simulink model "SeatHeaterapp"  (R2015a)
settings: Solver=FixedStepDiscrete  StartTime=0.0  StopTime=10.0  RelTol=1e-3
settings Model: Creator=Morya  LastModifiedBy=Morya
settings DataIOCC: SaveFormat=StructureWithTime
settings OptimizationCC: ZeroExternalMemoryAtStartup=off  ZeroInternalMemoryAtStartup=off  OptimizeModelRefInitCode=on  LifeSpan=1
settings ModelReferenceCC: ModelReferenceNumInstancesAllowed=Single
settings RTWCC: SystemTargetFile=autosar.tlc  GenCodeOnly=on  TemplateMakefile=ert_default_tmf  Description=AUTOSAR
settings CodeAppCC: IgnoreCustomStorageClasses=off
settings STFCustomTargetCC: GenerateSampleERTMain=off  ParMdlRefBuildCompliant=on  CompOptLevelCompliant=on  IncludeMdlTerminateFcn=off  CombineOutputUpdateFcns=on  SuppressErrorStatus=on  ERTFirstTimeCompliant=on  SupportNonFinite=off  SupportComplex=off  SupportContinuousTime=off  SupportVariableSizeSignals=off  AutosarCompliant=on  SystemTargetFile=autosar.tlc
settings ERTTargetCC: GenerateSampleERTMain=off  ParMdlRefBuildCompliant=on  CompOptLevelCompliant=on  IncludeMdlTerminateFcn=off  SuppressErrorStatus=on  ERTFirstTimeCompliant=on  SupportNonFinite=off  SupportComplex=off  SupportContinuousTime=off  SupportVariableSizeSignals=off  AutosarCompliant=on  ERTCustomFileTemplate=example_file_process.tlc

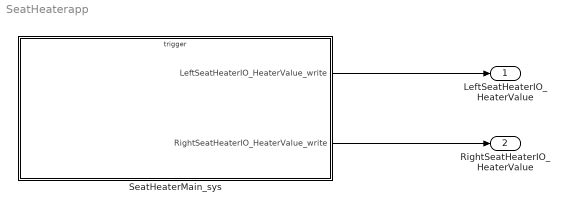
== system SeatHeaterapp ==
  SeatHeaterMain_sys : Subsystem
  LeftSeatHeaterIO_HeaterValue : Outport  OutDataTypeStr=Int32  PortDimensions=1
  RightSeatHeaterIO_HeaterValue : Outport  Port=2  OutDataTypeStr=Int32  PortDimensions=1
  wires:
  SeatHeaterMain_sys/1(LeftSeatHeaterIO_HeaterValue_write) -> LeftSeatHeaterIO_HeaterValue/1
  SeatHeaterMain_sys/2(RightSeatHeaterIO_HeaterValue_write) -> RightSeatHeaterIO_HeaterValue/1

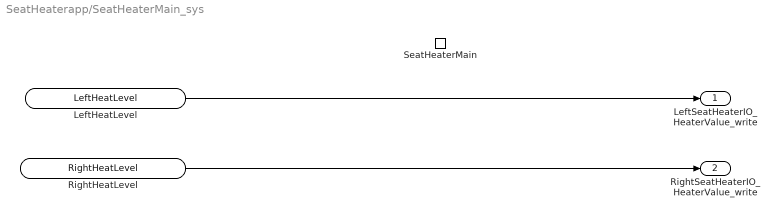
== system SeatHeaterapp/SeatHeaterMain_sys ==
  SeatHeaterMain : TriggerPort  TriggerType=function-call  IsSimulinkFunction=on  FunctionName=SeatHeaterMain
  LeftHeatLevel : ArgIn  OutDataTypeStr=Int32  ArgumentName=LeftHeatLevel
  RightHeatLevel : ArgIn  Port=2  OutDataTypeStr=Int32  ArgumentName=RightHeatLevel
  LeftSeatHeaterIO_HeaterValue_write : Outport
  RightSeatHeaterIO_HeaterValue_write : Outport  Port=2
  wires:
  LeftHeatLevel/1 -> LeftSeatHeaterIO_HeaterValue_write/1
  RightHeatLevel/1 -> RightSeatHeaterIO_HeaterValue_write/1
